simulink model "trifecta"  (R2021b)
settings: Solver=VariableStepAuto  StartTime=0.0  StopTime=10.0  RelTol=1e-3
libraries: sm_lib x2, vrlib x1
settings Model: Creator=gabom  LastModifiedBy=gabom

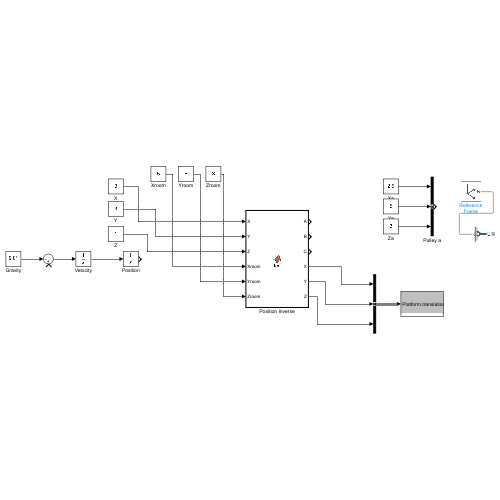
[thumbnail: Simulink's stored preview of the top-level diagram]
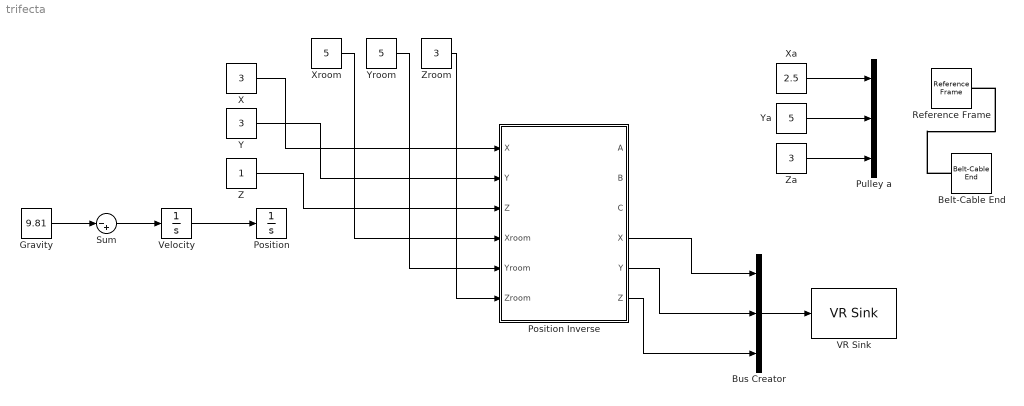
== system trifecta ==
  Belt-Cable End : sm_lib/Belts and Cables/Belt-Cable End
      settings: SourceProductBaseCode=MS
  Bus Creator : BusCreator  Inputs=3
  Gravity : Constant  Value=9.81
  Position : Integrator  InitialCondition=1.5
  Position Inverse : MATLAB Function  TreatAsAtomicUnit=on
  Pulley a : BusCreator  Inputs=3
  Reference Frame : sm_lib/Frames and Transforms/Reference Frame
  Sum : Sum  Inputs=|-+
  VR Sink : vrlib/VR Sink  InstantiateOnLoad=on  SampleTime=.001  ViewEnable=on  RemoteChange=off  RemoteView=off  FieldsWritten=Platform.translation.3.1.1.double  WorldFileName=trifectaSimulation.x3d  AutoView=off  VideoDimensions=[]  AllowVariableSize=off
  Velocity : Integrator
  X : Constant  Value=3
  Xa : Constant  Value=2.5
  Xroom : Constant  Value=5
  Y : Constant  Value=3
  Ya : Constant  Value=5
  Yroom : Constant  Value=5
  Z : Constant
  Za : Constant  Value=3
  Zroom : Constant  Value=3
  wires:
  Velocity/1 -> Position/1
  Sum/1 -> Velocity/1
  Gravity/1 -> Sum/1
  Xroom/1 -> Position Inverse/4(Xroom)
  Yroom/1 -> Position Inverse/5(Yroom)
  Zroom/1 -> Position Inverse/6(Zroom)
  Position Inverse/4(X) -> Bus Creator/1
  Position Inverse/5(Y) -> Bus Creator/2
  Position Inverse/6(Z) -> Bus Creator/3
  Bus Creator/1 -> VR Sink/1
  X/1 -> Position Inverse/1("X ")
  Y/1 -> Position Inverse/2("Y ")
  Z/1 -> Position Inverse/3("Z ")
  Xa/1 -> Pulley a/1
  Ya/1 -> Pulley a/2
  Za/1 -> Pulley a/3
  connections:
  Belt-Cable End/LConn1 -- Reference Frame/RConn1

== matlab function trifecta/Position Inverse ==
  data: X input; A output; Y input; Z input; B output; C output; Xroom input; Yroom input; Zroom input; X output; Y output; Z output
function [A, B, C, X, Y, Z] = fcn(X, Y, Z, Xroom, Yroom, Zroom)
% Determines the length of each cable to the requested position
% 
% Note than due to the platform's kinematic body, each mounting point is
% offset from the center of mass.

% floor limit
if(Y < 0)
    Y = 0;
end

theta = atan(Y/X);
thetaMax = atan(2*Yroom/Xroom);
% angle limit because of geometric work area
if(theta > thetaMax)
    theta = thetaMax;
end

% angle limit because of geometric work area
phi = atan(Y/(Xroom-X));
phiMax = atan(2*Yroom/Xroom);
if(phi > phiMax)
    phi = phiMax;
end

betaMax = 180 - phiMax - thetaMax;

B = sqrt(X^2 + Y^2 + Z^2)
C = sqrt((Xroom - X)^2 + Y^2 + Z^2)

gamma = phiMax - phi;
S = C*sin(gamma);
K = C*cos(gamma);

A = sqrt(S^2 + K^2 + Z^2)
